simulink model "dac_spi"  (R2022a)
settings: Solver=FixedStepDiscrete  StartTime=0.0  StopTime=1000/100e6  RelTol=1e-3
libraries: hdlsllib x152, simulink x1
settings Model: DataTypeOverride=Off  Creator=ts  LastModifiedBy=ts
settings SolverCC: AlgebraicLoopSolver=TrustRegion
settings DataIOCC: LimitDataPoints=on  SaveOutput=off  SaveTime=off
settings OptimizationCC: BlockReduction=off  ConditionallyExecuteInputs=off  DefaultParameterBehavior=Inlined  LifeSpan=inf
settings DebuggingCC: AlgebraicLoopMsg=error  SingleTaskRateTransMsg=error  UnconnectedInputMsg=warning  UnconnectedOutputMsg=warning  UnconnectedLineMsg=warning  AllowSymbolicDim=off  StrictBusMsg=ErrorOnBusTreatedAsVector  SFUnexpectedBacktrackingDiag=warning  SFNoUnconditionalDefaultTransitionDiag=warning  SFExecutionAtInitializationDiag=none  SFMachineParentedDataDiag=warning  ArithmeticOperatorsInVariantConditions=warning
settings HardwareCC: ProdBitPerPointer=32  ProdBitPerSizeT=32  ProdBitPerPtrDiffT=32  ProdLargestAtomicFloat=None  ProdIntDivRoundTo=Undefined  ProdEndianess=Unspecified  ProdWordSize=32  ProdHWDeviceType=ASIC/FPGA->ASIC/FPGA  ProdEqTarget=off
settings SFSimCC: SimUseLocalCustomCode=off  CustomCodeUndefinedFunction=UseInterfaceOnly
settings RTWCC: RTWUseLocalCustomCode=off
settings CodeAppCC: StateflowObjectComments=on
settings GRTTargetCC: TargetLangStandard=C89/C90 (ANSI)
settings ConfigComp: CovScope=ReferencedModels  CovMetricSettings=dw  CovSaveCumulativeToWorkspaceVar=on  CovSaveSingleToWorkspaceVar=on  CovExternalEMLEnable=off  CovSFcnEnable=off

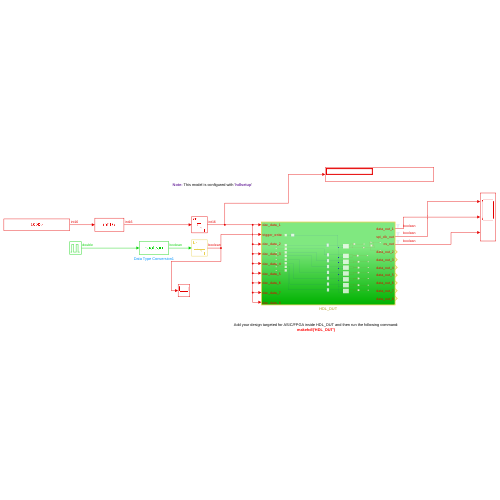
[thumbnail: Simulink's stored preview of the top-level diagram]
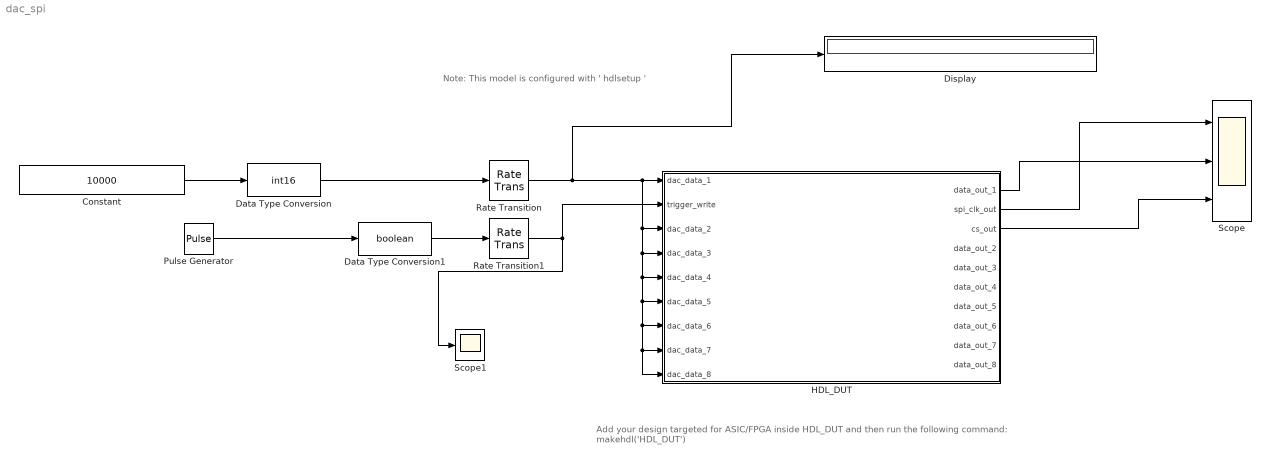
== system dac_spi ==
  note: Note: This model is configured with ' hdlsetup '
  note: Add your design targeted for ASIC/FPGA inside HDL_DUT and then run the following command:
      | makehdl('HDL_DUT')
  Constant : Constant  Value=10000  OutDataTypeStr=int16  SampleTime=1/100e6
  Data Type Conversion : DataTypeConversion  OutDataTypeStr=int16  SaturateOnIntegerOverflow=off  RndMeth=Floor
  Data Type Conversion1 : DataTypeConversion  OutDataTypeStr=boolean  SaturateOnIntegerOverflow=off  RndMeth=Floor
  Display : Display
      settings: Format=binary (Stored Integer)
  HDL_DUT : Subsystem  TreatAsAtomicUnit=on
  Pulse Generator : DiscretePulseGenerator  PulseType=Time based  Period=200/100e6  PulseWidth=10
  Rate Transition : RateTransition  OutPortSampleTime=1/100e6
  Rate Transition1 : RateTransition  OutPortSampleTime=1/100e6
  Scope : Scope  NumInputPorts=3
  Scope1 : Scope
  wires:
  Constant/1 -> Data Type Conversion/1
  HDL_DUT/1(data_out_1) -> Scope/2
  Data Type Conversion/1 -> Rate Transition/1
  Rate Transition/1 -> Display/1, HDL_DUT/9(dac_data_8), HDL_DUT/8(dac_data_7), HDL_DUT/7(dac_data_6), HDL_DUT/6(dac_data_5), HDL_DUT/5(dac_data_4), HDL_DUT/4(dac_data_3), HDL_DUT/3(dac_data_2), HDL_DUT/1(dac_data_1)
  HDL_DUT/3(cs_out) -> Scope/3
  HDL_DUT/2(spi_clk_out) -> Scope/1
  Rate Transition1/1 -> Scope1/1, HDL_DUT/2(trigger_write)
  Data Type Conversion1/1 -> Rate Transition1/1
  Pulse Generator/1 -> Data Type Conversion1/1

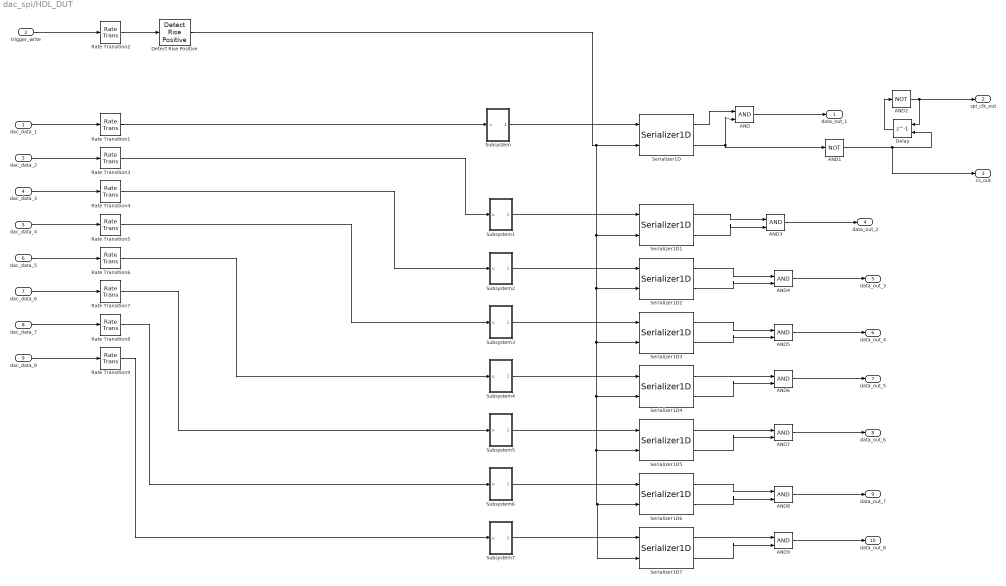
== system dac_spi/HDL_DUT ==
  dac_data_1 : Inport
  trigger_write : Inport  Port=2
  dac_data_2 : Inport  Port=3
  dac_data_3 : Inport  Port=4
  dac_data_4 : Inport  Port=5
  dac_data_5 : Inport  Port=6
  dac_data_6 : Inport  Port=7
  dac_data_7 : Inport  Port=8
  dac_data_8 : Inport  Port=9
  AND{,3..9} (8 alike) : Logic  IconShape=distinctive  AllPortsSameDT=off  OutDataTypeStr=boolean
  AND1 : Logic  Operator=NOT  IconShape=distinctive  AllPortsSameDT=off  OutDataTypeStr=boolean
  AND2 : Logic  Operator=NOT  IconShape=distinctive  AllPortsSameDT=off  OutDataTypeStr=boolean
  Delay : Delay  DelayLength=1  InitialCondition=1  ExternalReset=Level
      settings: InputPortMap=u0,r5
  Detect Rise Positive : simulink/Logic and Bit Operations/Detect Rise Positive  vinit=0  OutDataTypeStr=boolean
  Rate Transition{1..9} (9 alike) : RateTransition  OutPortSampleTime=32/100e6
  Serializer1D{,1..7} (8 alike) : hdlsllib/HDL Operations/Serializer1D  Ratio=32  IdleCycles=0  validIn=on  startOut=off  validOut=on  inputDataDimensions=-1  inputSampleTime=-1  inputSignalType=auto
      settings: SourceProductBaseCode=SL
  Subsystem : Subsystem
  Subsystem1 : Subsystem
  Subsystem2 : Subsystem
  Subsystem3 : Subsystem
  Subsystem4 : Subsystem
  Subsystem5 : Subsystem
  Subsystem6 : Subsystem
  Subsystem7 : Subsystem
  data_out_1 : Outport  VectorParamsAs1DForOutWhenUnconnected=off
  spi_clk_out : Outport  Port=2
  cs_out : Outport  Port=3
  data_out_2 : Outport  Port=4  VectorParamsAs1DForOutWhenUnconnected=off
  data_out_3 : Outport  Port=5  VectorParamsAs1DForOutWhenUnconnected=off
  data_out_4 : Outport  Port=6  VectorParamsAs1DForOutWhenUnconnected=off
  data_out_5 : Outport  Port=7  VectorParamsAs1DForOutWhenUnconnected=off
  data_out_6 : Outport  Port=8  VectorParamsAs1DForOutWhenUnconnected=off
  data_out_7 : Outport  Port=9  VectorParamsAs1DForOutWhenUnconnected=off
  data_out_8 : Outport  Port=10  VectorParamsAs1DForOutWhenUnconnected=off
  wires:
  AND/1 -> data_out_1/1
  Serializer1D/2 -> AND1/1, AND/2
  trigger_write/1 -> Rate Transition2/1
  dac_data_1/1 -> Rate Transition1/1
  Detect Rise Positive/1 -> Serializer1D7/2, Serializer1D6/2, Serializer1D5/2, Serializer1D4/2, Serializer1D3/2, Serializer1D2/2, Serializer1D1/2, Serializer1D/2
  Serializer1D/1 -> AND/1
  AND1/1 -> cs_out/1, Delay/2
  AND2/1 -> spi_clk_out/1, Delay/1
  Delay/1 -> AND2/1
  Rate Transition2/1 -> Detect Rise Positive/1
  Rate Transition1/1 -> Subsystem/1(u)
  Subsystem/1(Out1) -> Serializer1D/1
  Subsystem2/1(Out1) -> Serializer1D2/1
  Subsystem3/1(Out1) -> Serializer1D3/1
  Subsystem1/1(Out1) -> Serializer1D1/1
  dac_data_2/1 -> Rate Transition3/1
  dac_data_3/1 -> Rate Transition4/1
  dac_data_4/1 -> Rate Transition5/1
  dac_data_5/1 -> Rate Transition6/1
  dac_data_6/1 -> Rate Transition7/1
  dac_data_7/1 -> Rate Transition8/1
  dac_data_8/1 -> Rate Transition9/1
  Subsystem4/1(Out1) -> Serializer1D4/1
  Rate Transition3/1 -> Subsystem1/1(u)
  Rate Transition4/1 -> Subsystem2/1(u)
  Rate Transition5/1 -> Subsystem3/1(u)
  Rate Transition6/1 -> Subsystem4/1(u)
  Subsystem7/1(Out1) -> Serializer1D7/1
  Subsystem5/1(Out1) -> Serializer1D5/1
  Subsystem6/1(Out1) -> Serializer1D6/1
  Rate Transition7/1 -> Subsystem5/1(u)
  Rate Transition8/1 -> Subsystem6/1(u)
  Rate Transition9/1 -> Subsystem7/1(u)
  AND3/1 -> data_out_2/1
  Serializer1D1/1 -> AND3/1
  Serializer1D1/2 -> AND3/2
  AND4/1 -> data_out_3/1
  AND5/1 -> data_out_4/1
  AND6/1 -> data_out_5/1
  AND7/1 -> data_out_6/1
  AND8/1 -> data_out_7/1
  AND9/1 -> data_out_8/1
  Serializer1D2/1 -> AND4/1
  Serializer1D2/2 -> AND4/2
  Serializer1D3/1 -> AND5/1
  Serializer1D3/2 -> AND5/2
  Serializer1D4/1 -> AND6/1
  Serializer1D4/2 -> AND6/2
  Serializer1D5/1 -> AND7/1
  Serializer1D5/2 -> AND7/2
  Serializer1D6/1 -> AND8/1
  Serializer1D6/2 -> AND8/2
  Serializer1D7/1 -> AND9/1
  Serializer1D7/2 -> AND9/2

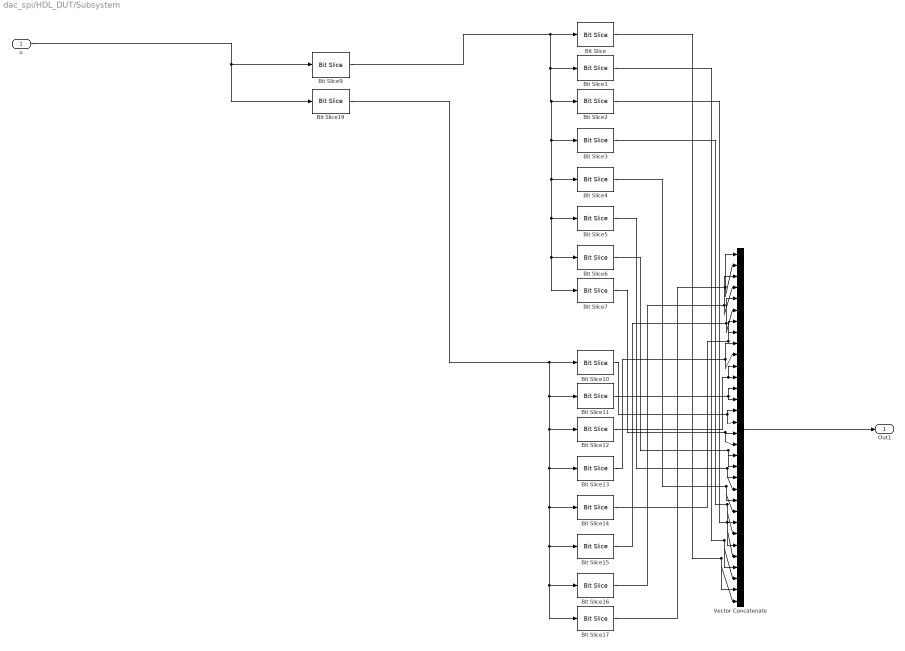
== system dac_spi/HDL_DUT/Subsystem ==
  u : Inport
  Bit Slice : hdlsllib/Logic and Bit Operations/Bit Slice  lidx=0  ridx=0
      settings: SourceProductBaseCode=SL
  Bit Slice1 : hdlsllib/Logic and Bit Operations/Bit Slice  lidx=1  ridx=1
      settings: SourceProductBaseCode=SL
  Bit Slice10 : hdlsllib/Logic and Bit Operations/Bit Slice  lidx=0  ridx=0
      settings: SourceProductBaseCode=SL
  Bit Slice11 : hdlsllib/Logic and Bit Operations/Bit Slice  lidx=1  ridx=1
      settings: SourceProductBaseCode=SL
  Bit Slice12 : hdlsllib/Logic and Bit Operations/Bit Slice  lidx=2  ridx=2
      settings: SourceProductBaseCode=SL
  Bit Slice13 : hdlsllib/Logic and Bit Operations/Bit Slice  lidx=3  ridx=3
      settings: SourceProductBaseCode=SL
  Bit Slice14 : hdlsllib/Logic and Bit Operations/Bit Slice  lidx=4  ridx=4
      settings: SourceProductBaseCode=SL
  Bit Slice15 : hdlsllib/Logic and Bit Operations/Bit Slice  lidx=5  ridx=5
      settings: SourceProductBaseCode=SL
  Bit Slice16 : hdlsllib/Logic and Bit Operations/Bit Slice  lidx=6  ridx=6
      settings: SourceProductBaseCode=SL
  Bit Slice17 : hdlsllib/Logic and Bit Operations/Bit Slice  lidx=7  ridx=7
      settings: SourceProductBaseCode=SL
  Bit Slice19 : hdlsllib/Logic and Bit Operations/Bit Slice  lidx=15  ridx=8
      settings: SourceProductBaseCode=SL
  Bit Slice2 : hdlsllib/Logic and Bit Operations/Bit Slice  lidx=2  ridx=2
      settings: SourceProductBaseCode=SL
  Bit Slice3 : hdlsllib/Logic and Bit Operations/Bit Slice  lidx=3  ridx=3
      settings: SourceProductBaseCode=SL
  Bit Slice4 : hdlsllib/Logic and Bit Operations/Bit Slice  lidx=4  ridx=4
      settings: SourceProductBaseCode=SL
  Bit Slice5 : hdlsllib/Logic and Bit Operations/Bit Slice  lidx=5  ridx=5
      settings: SourceProductBaseCode=SL
  Bit Slice6 : hdlsllib/Logic and Bit Operations/Bit Slice  lidx=6  ridx=6
      settings: SourceProductBaseCode=SL
  Bit Slice7 : hdlsllib/Logic and Bit Operations/Bit Slice  lidx=7  ridx=7
      settings: SourceProductBaseCode=SL
  Bit Slice9 : hdlsllib/Logic and Bit Operations/Bit Slice  lidx=7  ridx=0
      settings: SourceProductBaseCode=SL
  Vector Concatenate : Concatenate  NumInputs=32
  Out1 : Outport
  wires:
  Bit Slice10/1 -> Vector Concatenate/16, Vector Concatenate/15
  Bit Slice4/1 -> Vector Concatenate/24, Vector Concatenate/23
  Bit Slice6/1 -> Vector Concatenate/20, Vector Concatenate/19
  Bit Slice5/1 -> Vector Concatenate/22, Vector Concatenate/21
  u/1 -> Bit Slice19/1, Bit Slice9/1
  Bit Slice19/1 -> Bit Slice17/1, Bit Slice16/1, Bit Slice15/1, Bit Slice14/1, Bit Slice13/1, Bit Slice12/1, Bit Slice11/1, Bit Slice10/1
  Bit Slice11/1 -> Vector Concatenate/14, Vector Concatenate/13
  Bit Slice9/1 -> Bit Slice7/1, Bit Slice6/1, Bit Slice5/1, Bit Slice4/1, Bit Slice3/1, Bit Slice2/1, Bit Slice1/1, Bit Slice/1
  Bit Slice13/1 -> Vector Concatenate/10, Vector Concatenate/9
  Vector Concatenate/1 -> Out1/1
  Bit Slice7/1 -> Vector Concatenate/18, Vector Concatenate/17
  Bit Slice1/1 -> Vector Concatenate/30, Vector Concatenate/29
  Bit Slice/1 -> Vector Concatenate/32, Vector Concatenate/31
  Bit Slice17/1 -> Vector Concatenate/2, Vector Concatenate/1
  Bit Slice2/1 -> Vector Concatenate/28, Vector Concatenate/27
  Bit Slice12/1 -> Vector Concatenate/12, Vector Concatenate/11
  Bit Slice16/1 -> Vector Concatenate/4, Vector Concatenate/3
  Bit Slice14/1 -> Vector Concatenate/8, Vector Concatenate/7
  Bit Slice3/1 -> Vector Concatenate/26, Vector Concatenate/25
  Bit Slice15/1 -> Vector Concatenate/6, Vector Concatenate/5

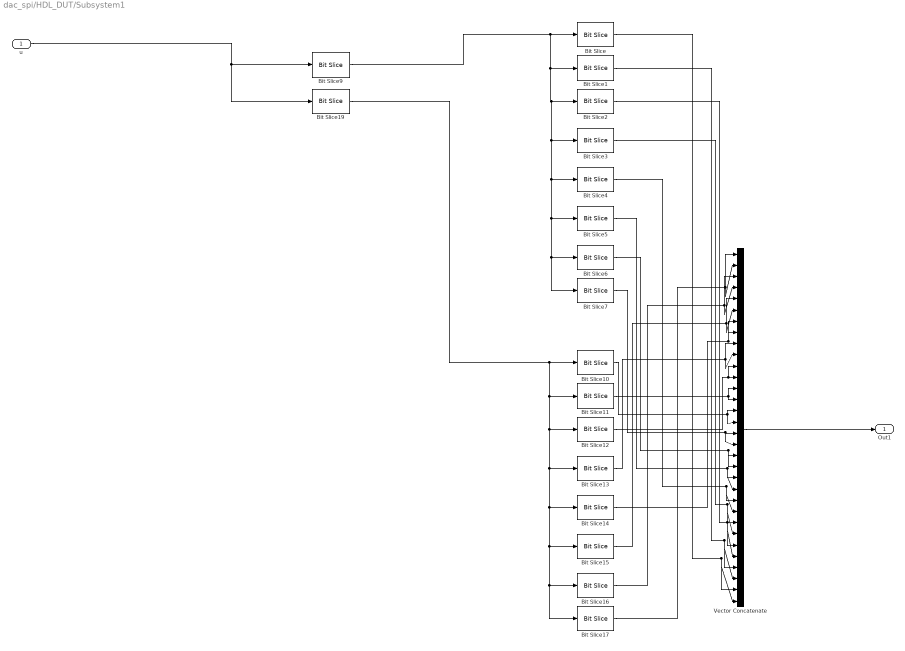
== system dac_spi/HDL_DUT/Subsystem1 ==
  u : Inport
  Bit Slice : hdlsllib/Logic and Bit Operations/Bit Slice  lidx=0  ridx=0
      settings: SourceProductBaseCode=SL
  Bit Slice1 : hdlsllib/Logic and Bit Operations/Bit Slice  lidx=1  ridx=1
      settings: SourceProductBaseCode=SL
  Bit Slice10 : hdlsllib/Logic and Bit Operations/Bit Slice  lidx=0  ridx=0
      settings: SourceProductBaseCode=SL
  Bit Slice11 : hdlsllib/Logic and Bit Operations/Bit Slice  lidx=1  ridx=1
      settings: SourceProductBaseCode=SL
  Bit Slice12 : hdlsllib/Logic and Bit Operations/Bit Slice  lidx=2  ridx=2
      settings: SourceProductBaseCode=SL
  Bit Slice13 : hdlsllib/Logic and Bit Operations/Bit Slice  lidx=3  ridx=3
      settings: SourceProductBaseCode=SL
  Bit Slice14 : hdlsllib/Logic and Bit Operations/Bit Slice  lidx=4  ridx=4
      settings: SourceProductBaseCode=SL
  Bit Slice15 : hdlsllib/Logic and Bit Operations/Bit Slice  lidx=5  ridx=5
      settings: SourceProductBaseCode=SL
  Bit Slice16 : hdlsllib/Logic and Bit Operations/Bit Slice  lidx=6  ridx=6
      settings: SourceProductBaseCode=SL
  Bit Slice17 : hdlsllib/Logic and Bit Operations/Bit Slice  lidx=7  ridx=7
      settings: SourceProductBaseCode=SL
  Bit Slice19 : hdlsllib/Logic and Bit Operations/Bit Slice  lidx=15  ridx=8
      settings: SourceProductBaseCode=SL
  Bit Slice2 : hdlsllib/Logic and Bit Operations/Bit Slice  lidx=2  ridx=2
      settings: SourceProductBaseCode=SL
  Bit Slice3 : hdlsllib/Logic and Bit Operations/Bit Slice  lidx=3  ridx=3
      settings: SourceProductBaseCode=SL
  Bit Slice4 : hdlsllib/Logic and Bit Operations/Bit Slice  lidx=4  ridx=4
      settings: SourceProductBaseCode=SL
  Bit Slice5 : hdlsllib/Logic and Bit Operations/Bit Slice  lidx=5  ridx=5
      settings: SourceProductBaseCode=SL
  Bit Slice6 : hdlsllib/Logic and Bit Operations/Bit Slice  lidx=6  ridx=6
      settings: SourceProductBaseCode=SL
  Bit Slice7 : hdlsllib/Logic and Bit Operations/Bit Slice  lidx=7  ridx=7
      settings: SourceProductBaseCode=SL
  Bit Slice9 : hdlsllib/Logic and Bit Operations/Bit Slice  lidx=7  ridx=0
      settings: SourceProductBaseCode=SL
  Vector Concatenate : Concatenate  NumInputs=32
  Out1 : Outport
  wires:
  Bit Slice15/1 -> Vector Concatenate/5, Vector Concatenate/6
  Bit Slice3/1 -> Vector Concatenate/25, Vector Concatenate/26
  Bit Slice14/1 -> Vector Concatenate/7, Vector Concatenate/8
  Bit Slice16/1 -> Vector Concatenate/3, Vector Concatenate/4
  Bit Slice12/1 -> Vector Concatenate/11, Vector Concatenate/12
  Bit Slice2/1 -> Vector Concatenate/27, Vector Concatenate/28
  Bit Slice17/1 -> Vector Concatenate/1, Vector Concatenate/2
  Bit Slice/1 -> Vector Concatenate/31, Vector Concatenate/32
  Bit Slice1/1 -> Vector Concatenate/29, Vector Concatenate/30
  Bit Slice7/1 -> Vector Concatenate/17, Vector Concatenate/18
  Vector Concatenate/1 -> Out1/1
  Bit Slice13/1 -> Vector Concatenate/9, Vector Concatenate/10
  Bit Slice9/1 -> Bit Slice/1, Bit Slice1/1, Bit Slice2/1, Bit Slice3/1, Bit Slice4/1, Bit Slice5/1, Bit Slice6/1, Bit Slice7/1
  Bit Slice11/1 -> Vector Concatenate/13, Vector Concatenate/14
  Bit Slice19/1 -> Bit Slice10/1, Bit Slice11/1, Bit Slice12/1, Bit Slice13/1, Bit Slice14/1, Bit Slice15/1, Bit Slice16/1, Bit Slice17/1
  u/1 -> Bit Slice9/1, Bit Slice19/1
  Bit Slice5/1 -> Vector Concatenate/21, Vector Concatenate/22
  Bit Slice6/1 -> Vector Concatenate/19, Vector Concatenate/20
  Bit Slice4/1 -> Vector Concatenate/23, Vector Concatenate/24
  Bit Slice10/1 -> Vector Concatenate/15, Vector Concatenate/16

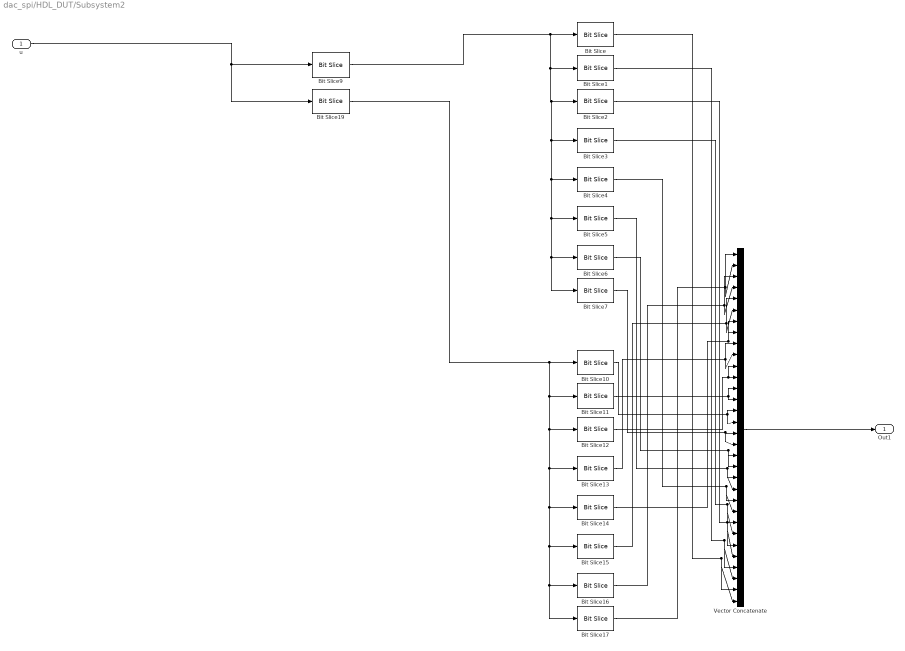
== system dac_spi/HDL_DUT/Subsystem2 ==
  u : Inport
  Bit Slice : hdlsllib/Logic and Bit Operations/Bit Slice  lidx=0  ridx=0
      settings: SourceProductBaseCode=SL
  Bit Slice1 : hdlsllib/Logic and Bit Operations/Bit Slice  lidx=1  ridx=1
      settings: SourceProductBaseCode=SL
  Bit Slice10 : hdlsllib/Logic and Bit Operations/Bit Slice  lidx=0  ridx=0
      settings: SourceProductBaseCode=SL
  Bit Slice11 : hdlsllib/Logic and Bit Operations/Bit Slice  lidx=1  ridx=1
      settings: SourceProductBaseCode=SL
  Bit Slice12 : hdlsllib/Logic and Bit Operations/Bit Slice  lidx=2  ridx=2
      settings: SourceProductBaseCode=SL
  Bit Slice13 : hdlsllib/Logic and Bit Operations/Bit Slice  lidx=3  ridx=3
      settings: SourceProductBaseCode=SL
  Bit Slice14 : hdlsllib/Logic and Bit Operations/Bit Slice  lidx=4  ridx=4
      settings: SourceProductBaseCode=SL
  Bit Slice15 : hdlsllib/Logic and Bit Operations/Bit Slice  lidx=5  ridx=5
      settings: SourceProductBaseCode=SL
  Bit Slice16 : hdlsllib/Logic and Bit Operations/Bit Slice  lidx=6  ridx=6
      settings: SourceProductBaseCode=SL
  Bit Slice17 : hdlsllib/Logic and Bit Operations/Bit Slice  lidx=7  ridx=7
      settings: SourceProductBaseCode=SL
  Bit Slice19 : hdlsllib/Logic and Bit Operations/Bit Slice  lidx=15  ridx=8
      settings: SourceProductBaseCode=SL
  Bit Slice2 : hdlsllib/Logic and Bit Operations/Bit Slice  lidx=2  ridx=2
      settings: SourceProductBaseCode=SL
  Bit Slice3 : hdlsllib/Logic and Bit Operations/Bit Slice  lidx=3  ridx=3
      settings: SourceProductBaseCode=SL
  Bit Slice4 : hdlsllib/Logic and Bit Operations/Bit Slice  lidx=4  ridx=4
      settings: SourceProductBaseCode=SL
  Bit Slice5 : hdlsllib/Logic and Bit Operations/Bit Slice  lidx=5  ridx=5
      settings: SourceProductBaseCode=SL
  Bit Slice6 : hdlsllib/Logic and Bit Operations/Bit Slice  lidx=6  ridx=6
      settings: SourceProductBaseCode=SL
  Bit Slice7 : hdlsllib/Logic and Bit Operations/Bit Slice  lidx=7  ridx=7
      settings: SourceProductBaseCode=SL
  Bit Slice9 : hdlsllib/Logic and Bit Operations/Bit Slice  lidx=7  ridx=0
      settings: SourceProductBaseCode=SL
  Vector Concatenate : Concatenate  NumInputs=32
  Out1 : Outport
  wires:
  Bit Slice10/1 -> Vector Concatenate/16, Vector Concatenate/15
  Bit Slice4/1 -> Vector Concatenate/24, Vector Concatenate/23
  Bit Slice6/1 -> Vector Concatenate/20, Vector Concatenate/19
  Bit Slice5/1 -> Vector Concatenate/22, Vector Concatenate/21
  u/1 -> Bit Slice19/1, Bit Slice9/1
  Bit Slice19/1 -> Bit Slice17/1, Bit Slice16/1, Bit Slice15/1, Bit Slice14/1, Bit Slice13/1, Bit Slice12/1, Bit Slice11/1, Bit Slice10/1
  Bit Slice11/1 -> Vector Concatenate/14, Vector Concatenate/13
  Bit Slice9/1 -> Bit Slice7/1, Bit Slice6/1, Bit Slice5/1, Bit Slice4/1, Bit Slice3/1, Bit Slice2/1, Bit Slice1/1, Bit Slice/1
  Bit Slice13/1 -> Vector Concatenate/10, Vector Concatenate/9
  Vector Concatenate/1 -> Out1/1
  Bit Slice7/1 -> Vector Concatenate/18, Vector Concatenate/17
  Bit Slice1/1 -> Vector Concatenate/30, Vector Concatenate/29
  Bit Slice/1 -> Vector Concatenate/32, Vector Concatenate/31
  Bit Slice17/1 -> Vector Concatenate/2, Vector Concatenate/1
  Bit Slice2/1 -> Vector Concatenate/28, Vector Concatenate/27
  Bit Slice12/1 -> Vector Concatenate/12, Vector Concatenate/11
  Bit Slice16/1 -> Vector Concatenate/4, Vector Concatenate/3
  Bit Slice14/1 -> Vector Concatenate/8, Vector Concatenate/7
  Bit Slice3/1 -> Vector Concatenate/26, Vector Concatenate/25
  Bit Slice15/1 -> Vector Concatenate/6, Vector Concatenate/5

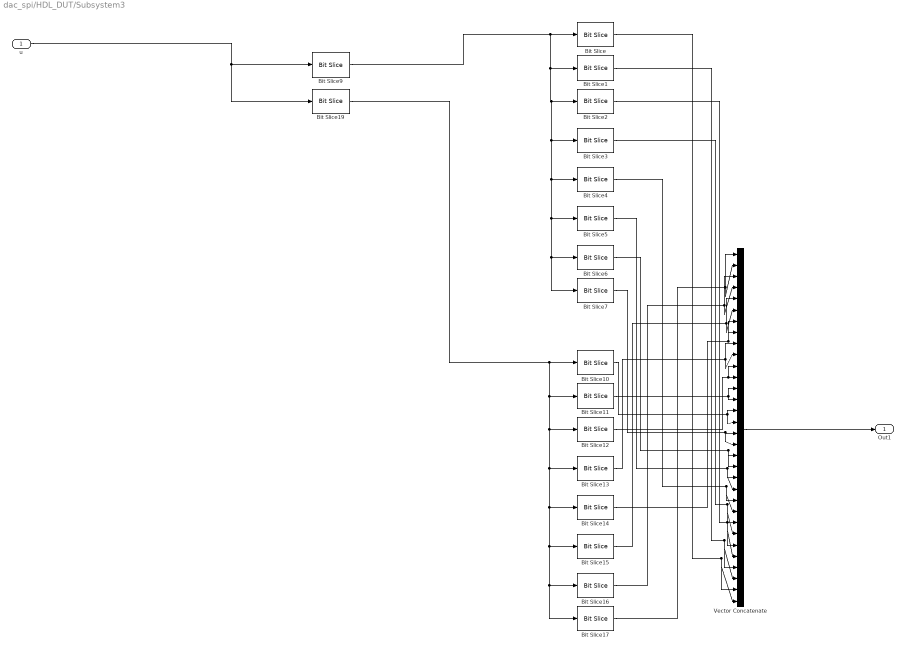
== system dac_spi/HDL_DUT/Subsystem3 ==
  u : Inport
  Bit Slice : hdlsllib/Logic and Bit Operations/Bit Slice  lidx=0  ridx=0
      settings: SourceProductBaseCode=SL
  Bit Slice1 : hdlsllib/Logic and Bit Operations/Bit Slice  lidx=1  ridx=1
      settings: SourceProductBaseCode=SL
  Bit Slice10 : hdlsllib/Logic and Bit Operations/Bit Slice  lidx=0  ridx=0
      settings: SourceProductBaseCode=SL
  Bit Slice11 : hdlsllib/Logic and Bit Operations/Bit Slice  lidx=1  ridx=1
      settings: SourceProductBaseCode=SL
  Bit Slice12 : hdlsllib/Logic and Bit Operations/Bit Slice  lidx=2  ridx=2
      settings: SourceProductBaseCode=SL
  Bit Slice13 : hdlsllib/Logic and Bit Operations/Bit Slice  lidx=3  ridx=3
      settings: SourceProductBaseCode=SL
  Bit Slice14 : hdlsllib/Logic and Bit Operations/Bit Slice  lidx=4  ridx=4
      settings: SourceProductBaseCode=SL
  Bit Slice15 : hdlsllib/Logic and Bit Operations/Bit Slice  lidx=5  ridx=5
      settings: SourceProductBaseCode=SL
  Bit Slice16 : hdlsllib/Logic and Bit Operations/Bit Slice  lidx=6  ridx=6
      settings: SourceProductBaseCode=SL
  Bit Slice17 : hdlsllib/Logic and Bit Operations/Bit Slice  lidx=7  ridx=7
      settings: SourceProductBaseCode=SL
  Bit Slice19 : hdlsllib/Logic and Bit Operations/Bit Slice  lidx=15  ridx=8
      settings: SourceProductBaseCode=SL
  Bit Slice2 : hdlsllib/Logic and Bit Operations/Bit Slice  lidx=2  ridx=2
      settings: SourceProductBaseCode=SL
  Bit Slice3 : hdlsllib/Logic and Bit Operations/Bit Slice  lidx=3  ridx=3
      settings: SourceProductBaseCode=SL
  Bit Slice4 : hdlsllib/Logic and Bit Operations/Bit Slice  lidx=4  ridx=4
      settings: SourceProductBaseCode=SL
  Bit Slice5 : hdlsllib/Logic and Bit Operations/Bit Slice  lidx=5  ridx=5
      settings: SourceProductBaseCode=SL
  Bit Slice6 : hdlsllib/Logic and Bit Operations/Bit Slice  lidx=6  ridx=6
      settings: SourceProductBaseCode=SL
  Bit Slice7 : hdlsllib/Logic and Bit Operations/Bit Slice  lidx=7  ridx=7
      settings: SourceProductBaseCode=SL
  Bit Slice9 : hdlsllib/Logic and Bit Operations/Bit Slice  lidx=7  ridx=0
      settings: SourceProductBaseCode=SL
  Vector Concatenate : Concatenate  NumInputs=32
  Out1 : Outport
  wires:
  Bit Slice15/1 -> Vector Concatenate/5, Vector Concatenate/6
  Bit Slice3/1 -> Vector Concatenate/25, Vector Concatenate/26
  Bit Slice14/1 -> Vector Concatenate/7, Vector Concatenate/8
  Bit Slice16/1 -> Vector Concatenate/3, Vector Concatenate/4
  Bit Slice12/1 -> Vector Concatenate/11, Vector Concatenate/12
  Bit Slice2/1 -> Vector Concatenate/27, Vector Concatenate/28
  Bit Slice17/1 -> Vector Concatenate/1, Vector Concatenate/2
  Bit Slice/1 -> Vector Concatenate/31, Vector Concatenate/32
  Bit Slice1/1 -> Vector Concatenate/29, Vector Concatenate/30
  Bit Slice7/1 -> Vector Concatenate/17, Vector Concatenate/18
  Vector Concatenate/1 -> Out1/1
  Bit Slice13/1 -> Vector Concatenate/9, Vector Concatenate/10
  Bit Slice9/1 -> Bit Slice/1, Bit Slice1/1, Bit Slice2/1, Bit Slice3/1, Bit Slice4/1, Bit Slice5/1, Bit Slice6/1, Bit Slice7/1
  Bit Slice11/1 -> Vector Concatenate/13, Vector Concatenate/14
  Bit Slice19/1 -> Bit Slice10/1, Bit Slice11/1, Bit Slice12/1, Bit Slice13/1, Bit Slice14/1, Bit Slice15/1, Bit Slice16/1, Bit Slice17/1
  u/1 -> Bit Slice9/1, Bit Slice19/1
  Bit Slice5/1 -> Vector Concatenate/21, Vector Concatenate/22
  Bit Slice6/1 -> Vector Concatenate/19, Vector Concatenate/20
  Bit Slice4/1 -> Vector Concatenate/23, Vector Concatenate/24
  Bit Slice10/1 -> Vector Concatenate/15, Vector Concatenate/16

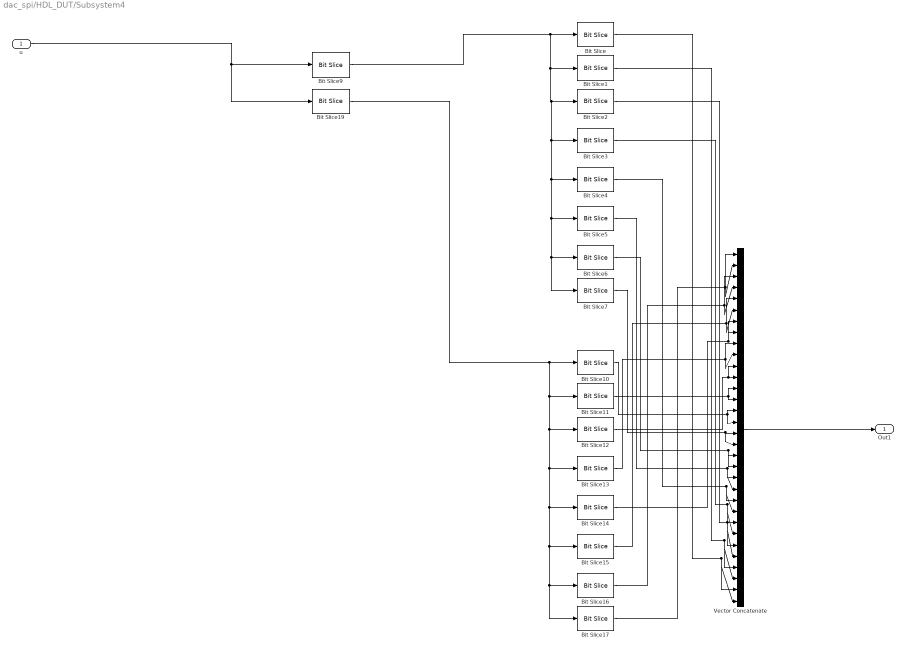
== system dac_spi/HDL_DUT/Subsystem4 ==
  u : Inport
  Bit Slice : hdlsllib/Logic and Bit Operations/Bit Slice  lidx=0  ridx=0
      settings: SourceProductBaseCode=SL
  Bit Slice1 : hdlsllib/Logic and Bit Operations/Bit Slice  lidx=1  ridx=1
      settings: SourceProductBaseCode=SL
  Bit Slice10 : hdlsllib/Logic and Bit Operations/Bit Slice  lidx=0  ridx=0
      settings: SourceProductBaseCode=SL
  Bit Slice11 : hdlsllib/Logic and Bit Operations/Bit Slice  lidx=1  ridx=1
      settings: SourceProductBaseCode=SL
  Bit Slice12 : hdlsllib/Logic and Bit Operations/Bit Slice  lidx=2  ridx=2
      settings: SourceProductBaseCode=SL
  Bit Slice13 : hdlsllib/Logic and Bit Operations/Bit Slice  lidx=3  ridx=3
      settings: SourceProductBaseCode=SL
  Bit Slice14 : hdlsllib/Logic and Bit Operations/Bit Slice  lidx=4  ridx=4
      settings: SourceProductBaseCode=SL
  Bit Slice15 : hdlsllib/Logic and Bit Operations/Bit Slice  lidx=5  ridx=5
      settings: SourceProductBaseCode=SL
  Bit Slice16 : hdlsllib/Logic and Bit Operations/Bit Slice  lidx=6  ridx=6
      settings: SourceProductBaseCode=SL
  Bit Slice17 : hdlsllib/Logic and Bit Operations/Bit Slice  lidx=7  ridx=7
      settings: SourceProductBaseCode=SL
  Bit Slice19 : hdlsllib/Logic and Bit Operations/Bit Slice  lidx=15  ridx=8
      settings: SourceProductBaseCode=SL
  Bit Slice2 : hdlsllib/Logic and Bit Operations/Bit Slice  lidx=2  ridx=2
      settings: SourceProductBaseCode=SL
  Bit Slice3 : hdlsllib/Logic and Bit Operations/Bit Slice  lidx=3  ridx=3
      settings: SourceProductBaseCode=SL
  Bit Slice4 : hdlsllib/Logic and Bit Operations/Bit Slice  lidx=4  ridx=4
      settings: SourceProductBaseCode=SL
  Bit Slice5 : hdlsllib/Logic and Bit Operations/Bit Slice  lidx=5  ridx=5
      settings: SourceProductBaseCode=SL
  Bit Slice6 : hdlsllib/Logic and Bit Operations/Bit Slice  lidx=6  ridx=6
      settings: SourceProductBaseCode=SL
  Bit Slice7 : hdlsllib/Logic and Bit Operations/Bit Slice  lidx=7  ridx=7
      settings: SourceProductBaseCode=SL
  Bit Slice9 : hdlsllib/Logic and Bit Operations/Bit Slice  lidx=7  ridx=0
      settings: SourceProductBaseCode=SL
  Vector Concatenate : Concatenate  NumInputs=32
  Out1 : Outport
  wires:
  Bit Slice15/1 -> Vector Concatenate/5, Vector Concatenate/6
  Bit Slice3/1 -> Vector Concatenate/25, Vector Concatenate/26
  Bit Slice14/1 -> Vector Concatenate/7, Vector Concatenate/8
  Bit Slice16/1 -> Vector Concatenate/3, Vector Concatenate/4
  Bit Slice12/1 -> Vector Concatenate/11, Vector Concatenate/12
  Bit Slice2/1 -> Vector Concatenate/27, Vector Concatenate/28
  Bit Slice17/1 -> Vector Concatenate/1, Vector Concatenate/2
  Bit Slice/1 -> Vector Concatenate/31, Vector Concatenate/32
  Bit Slice1/1 -> Vector Concatenate/29, Vector Concatenate/30
  Bit Slice7/1 -> Vector Concatenate/17, Vector Concatenate/18
  Vector Concatenate/1 -> Out1/1
  Bit Slice13/1 -> Vector Concatenate/9, Vector Concatenate/10
  Bit Slice9/1 -> Bit Slice/1, Bit Slice1/1, Bit Slice2/1, Bit Slice3/1, Bit Slice4/1, Bit Slice5/1, Bit Slice6/1, Bit Slice7/1
  Bit Slice11/1 -> Vector Concatenate/13, Vector Concatenate/14
  Bit Slice19/1 -> Bit Slice10/1, Bit Slice11/1, Bit Slice12/1, Bit Slice13/1, Bit Slice14/1, Bit Slice15/1, Bit Slice16/1, Bit Slice17/1
  u/1 -> Bit Slice9/1, Bit Slice19/1
  Bit Slice5/1 -> Vector Concatenate/21, Vector Concatenate/22
  Bit Slice6/1 -> Vector Concatenate/19, Vector Concatenate/20
  Bit Slice4/1 -> Vector Concatenate/23, Vector Concatenate/24
  Bit Slice10/1 -> Vector Concatenate/15, Vector Concatenate/16

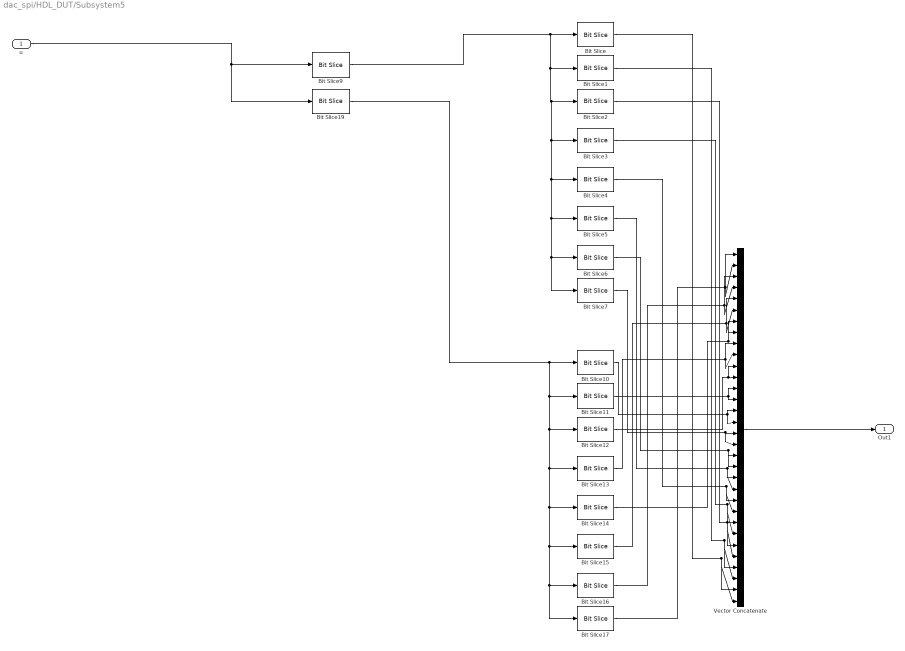
== system dac_spi/HDL_DUT/Subsystem5 ==
  u : Inport
  Bit Slice : hdlsllib/Logic and Bit Operations/Bit Slice  lidx=0  ridx=0
      settings: SourceProductBaseCode=SL
  Bit Slice1 : hdlsllib/Logic and Bit Operations/Bit Slice  lidx=1  ridx=1
      settings: SourceProductBaseCode=SL
  Bit Slice10 : hdlsllib/Logic and Bit Operations/Bit Slice  lidx=0  ridx=0
      settings: SourceProductBaseCode=SL
  Bit Slice11 : hdlsllib/Logic and Bit Operations/Bit Slice  lidx=1  ridx=1
      settings: SourceProductBaseCode=SL
  Bit Slice12 : hdlsllib/Logic and Bit Operations/Bit Slice  lidx=2  ridx=2
      settings: SourceProductBaseCode=SL
  Bit Slice13 : hdlsllib/Logic and Bit Operations/Bit Slice  lidx=3  ridx=3
      settings: SourceProductBaseCode=SL
  Bit Slice14 : hdlsllib/Logic and Bit Operations/Bit Slice  lidx=4  ridx=4
      settings: SourceProductBaseCode=SL
  Bit Slice15 : hdlsllib/Logic and Bit Operations/Bit Slice  lidx=5  ridx=5
      settings: SourceProductBaseCode=SL
  Bit Slice16 : hdlsllib/Logic and Bit Operations/Bit Slice  lidx=6  ridx=6
      settings: SourceProductBaseCode=SL
  Bit Slice17 : hdlsllib/Logic and Bit Operations/Bit Slice  lidx=7  ridx=7
      settings: SourceProductBaseCode=SL
  Bit Slice19 : hdlsllib/Logic and Bit Operations/Bit Slice  lidx=15  ridx=8
      settings: SourceProductBaseCode=SL
  Bit Slice2 : hdlsllib/Logic and Bit Operations/Bit Slice  lidx=2  ridx=2
      settings: SourceProductBaseCode=SL
  Bit Slice3 : hdlsllib/Logic and Bit Operations/Bit Slice  lidx=3  ridx=3
      settings: SourceProductBaseCode=SL
  Bit Slice4 : hdlsllib/Logic and Bit Operations/Bit Slice  lidx=4  ridx=4
      settings: SourceProductBaseCode=SL
  Bit Slice5 : hdlsllib/Logic and Bit Operations/Bit Slice  lidx=5  ridx=5
      settings: SourceProductBaseCode=SL
  Bit Slice6 : hdlsllib/Logic and Bit Operations/Bit Slice  lidx=6  ridx=6
      settings: SourceProductBaseCode=SL
  Bit Slice7 : hdlsllib/Logic and Bit Operations/Bit Slice  lidx=7  ridx=7
      settings: SourceProductBaseCode=SL
  Bit Slice9 : hdlsllib/Logic and Bit Operations/Bit Slice  lidx=7  ridx=0
      settings: SourceProductBaseCode=SL
  Vector Concatenate : Concatenate  NumInputs=32
  Out1 : Outport
  wires:
  Bit Slice10/1 -> Vector Concatenate/16, Vector Concatenate/15
  Bit Slice4/1 -> Vector Concatenate/24, Vector Concatenate/23
  Bit Slice6/1 -> Vector Concatenate/20, Vector Concatenate/19
  Bit Slice5/1 -> Vector Concatenate/22, Vector Concatenate/21
  u/1 -> Bit Slice19/1, Bit Slice9/1
  Bit Slice19/1 -> Bit Slice17/1, Bit Slice16/1, Bit Slice15/1, Bit Slice14/1, Bit Slice13/1, Bit Slice12/1, Bit Slice11/1, Bit Slice10/1
  Bit Slice11/1 -> Vector Concatenate/14, Vector Concatenate/13
  Bit Slice9/1 -> Bit Slice7/1, Bit Slice6/1, Bit Slice5/1, Bit Slice4/1, Bit Slice3/1, Bit Slice2/1, Bit Slice1/1, Bit Slice/1
  Bit Slice13/1 -> Vector Concatenate/10, Vector Concatenate/9
  Vector Concatenate/1 -> Out1/1
  Bit Slice7/1 -> Vector Concatenate/18, Vector Concatenate/17
  Bit Slice1/1 -> Vector Concatenate/30, Vector Concatenate/29
  Bit Slice/1 -> Vector Concatenate/32, Vector Concatenate/31
  Bit Slice17/1 -> Vector Concatenate/2, Vector Concatenate/1
  Bit Slice2/1 -> Vector Concatenate/28, Vector Concatenate/27
  Bit Slice12/1 -> Vector Concatenate/12, Vector Concatenate/11
  Bit Slice16/1 -> Vector Concatenate/4, Vector Concatenate/3
  Bit Slice14/1 -> Vector Concatenate/8, Vector Concatenate/7
  Bit Slice3/1 -> Vector Concatenate/26, Vector Concatenate/25
  Bit Slice15/1 -> Vector Concatenate/6, Vector Concatenate/5

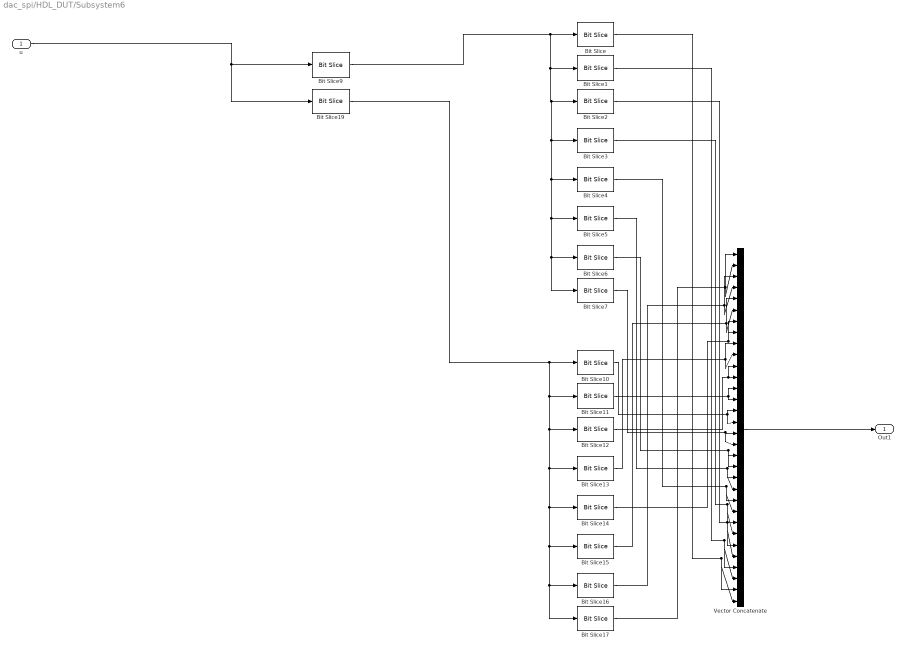
== system dac_spi/HDL_DUT/Subsystem6 ==
  u : Inport
  Bit Slice : hdlsllib/Logic and Bit Operations/Bit Slice  lidx=0  ridx=0
      settings: SourceProductBaseCode=SL
  Bit Slice1 : hdlsllib/Logic and Bit Operations/Bit Slice  lidx=1  ridx=1
      settings: SourceProductBaseCode=SL
  Bit Slice10 : hdlsllib/Logic and Bit Operations/Bit Slice  lidx=0  ridx=0
      settings: SourceProductBaseCode=SL
  Bit Slice11 : hdlsllib/Logic and Bit Operations/Bit Slice  lidx=1  ridx=1
      settings: SourceProductBaseCode=SL
  Bit Slice12 : hdlsllib/Logic and Bit Operations/Bit Slice  lidx=2  ridx=2
      settings: SourceProductBaseCode=SL
  Bit Slice13 : hdlsllib/Logic and Bit Operations/Bit Slice  lidx=3  ridx=3
      settings: SourceProductBaseCode=SL
  Bit Slice14 : hdlsllib/Logic and Bit Operations/Bit Slice  lidx=4  ridx=4
      settings: SourceProductBaseCode=SL
  Bit Slice15 : hdlsllib/Logic and Bit Operations/Bit Slice  lidx=5  ridx=5
      settings: SourceProductBaseCode=SL
  Bit Slice16 : hdlsllib/Logic and Bit Operations/Bit Slice  lidx=6  ridx=6
      settings: SourceProductBaseCode=SL
  Bit Slice17 : hdlsllib/Logic and Bit Operations/Bit Slice  lidx=7  ridx=7
      settings: SourceProductBaseCode=SL
  Bit Slice19 : hdlsllib/Logic and Bit Operations/Bit Slice  lidx=15  ridx=8
      settings: SourceProductBaseCode=SL
  Bit Slice2 : hdlsllib/Logic and Bit Operations/Bit Slice  lidx=2  ridx=2
      settings: SourceProductBaseCode=SL
  Bit Slice3 : hdlsllib/Logic and Bit Operations/Bit Slice  lidx=3  ridx=3
      settings: SourceProductBaseCode=SL
  Bit Slice4 : hdlsllib/Logic and Bit Operations/Bit Slice  lidx=4  ridx=4
      settings: SourceProductBaseCode=SL
  Bit Slice5 : hdlsllib/Logic and Bit Operations/Bit Slice  lidx=5  ridx=5
      settings: SourceProductBaseCode=SL
  Bit Slice6 : hdlsllib/Logic and Bit Operations/Bit Slice  lidx=6  ridx=6
      settings: SourceProductBaseCode=SL
  Bit Slice7 : hdlsllib/Logic and Bit Operations/Bit Slice  lidx=7  ridx=7
      settings: SourceProductBaseCode=SL
  Bit Slice9 : hdlsllib/Logic and Bit Operations/Bit Slice  lidx=7  ridx=0
      settings: SourceProductBaseCode=SL
  Vector Concatenate : Concatenate  NumInputs=32
  Out1 : Outport
  wires:
  Bit Slice15/1 -> Vector Concatenate/5, Vector Concatenate/6
  Bit Slice3/1 -> Vector Concatenate/25, Vector Concatenate/26
  Bit Slice14/1 -> Vector Concatenate/7, Vector Concatenate/8
  Bit Slice16/1 -> Vector Concatenate/3, Vector Concatenate/4
  Bit Slice12/1 -> Vector Concatenate/11, Vector Concatenate/12
  Bit Slice2/1 -> Vector Concatenate/27, Vector Concatenate/28
  Bit Slice17/1 -> Vector Concatenate/1, Vector Concatenate/2
  Bit Slice/1 -> Vector Concatenate/31, Vector Concatenate/32
  Bit Slice1/1 -> Vector Concatenate/29, Vector Concatenate/30
  Bit Slice7/1 -> Vector Concatenate/17, Vector Concatenate/18
  Vector Concatenate/1 -> Out1/1
  Bit Slice13/1 -> Vector Concatenate/9, Vector Concatenate/10
  Bit Slice9/1 -> Bit Slice/1, Bit Slice1/1, Bit Slice2/1, Bit Slice3/1, Bit Slice4/1, Bit Slice5/1, Bit Slice6/1, Bit Slice7/1
  Bit Slice11/1 -> Vector Concatenate/13, Vector Concatenate/14
  Bit Slice19/1 -> Bit Slice10/1, Bit Slice11/1, Bit Slice12/1, Bit Slice13/1, Bit Slice14/1, Bit Slice15/1, Bit Slice16/1, Bit Slice17/1
  u/1 -> Bit Slice9/1, Bit Slice19/1
  Bit Slice5/1 -> Vector Concatenate/21, Vector Concatenate/22
  Bit Slice6/1 -> Vector Concatenate/19, Vector Concatenate/20
  Bit Slice4/1 -> Vector Concatenate/23, Vector Concatenate/24
  Bit Slice10/1 -> Vector Concatenate/15, Vector Concatenate/16

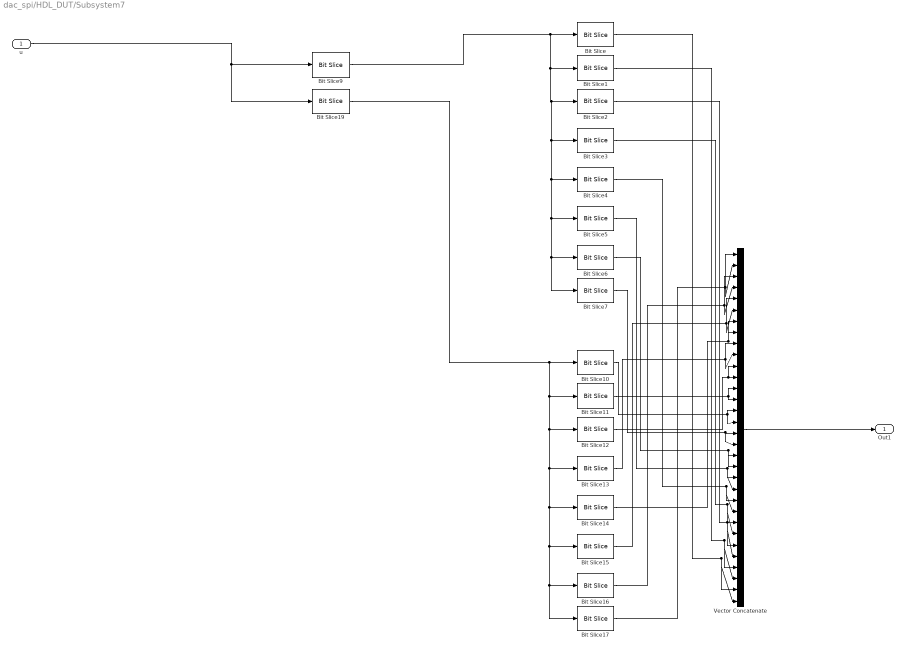
== system dac_spi/HDL_DUT/Subsystem7 ==
  u : Inport
  Bit Slice : hdlsllib/Logic and Bit Operations/Bit Slice  lidx=0  ridx=0
      settings: SourceProductBaseCode=SL
  Bit Slice1 : hdlsllib/Logic and Bit Operations/Bit Slice  lidx=1  ridx=1
      settings: SourceProductBaseCode=SL
  Bit Slice10 : hdlsllib/Logic and Bit Operations/Bit Slice  lidx=0  ridx=0
      settings: SourceProductBaseCode=SL
  Bit Slice11 : hdlsllib/Logic and Bit Operations/Bit Slice  lidx=1  ridx=1
      settings: SourceProductBaseCode=SL
  Bit Slice12 : hdlsllib/Logic and Bit Operations/Bit Slice  lidx=2  ridx=2
      settings: SourceProductBaseCode=SL
  Bit Slice13 : hdlsllib/Logic and Bit Operations/Bit Slice  lidx=3  ridx=3
      settings: SourceProductBaseCode=SL
  Bit Slice14 : hdlsllib/Logic and Bit Operations/Bit Slice  lidx=4  ridx=4
      settings: SourceProductBaseCode=SL
  Bit Slice15 : hdlsllib/Logic and Bit Operations/Bit Slice  lidx=5  ridx=5
      settings: SourceProductBaseCode=SL
  Bit Slice16 : hdlsllib/Logic and Bit Operations/Bit Slice  lidx=6  ridx=6
      settings: SourceProductBaseCode=SL
  Bit Slice17 : hdlsllib/Logic and Bit Operations/Bit Slice  lidx=7  ridx=7
      settings: SourceProductBaseCode=SL
  Bit Slice19 : hdlsllib/Logic and Bit Operations/Bit Slice  lidx=15  ridx=8
      settings: SourceProductBaseCode=SL
  Bit Slice2 : hdlsllib/Logic and Bit Operations/Bit Slice  lidx=2  ridx=2
      settings: SourceProductBaseCode=SL
  Bit Slice3 : hdlsllib/Logic and Bit Operations/Bit Slice  lidx=3  ridx=3
      settings: SourceProductBaseCode=SL
  Bit Slice4 : hdlsllib/Logic and Bit Operations/Bit Slice  lidx=4  ridx=4
      settings: SourceProductBaseCode=SL
  Bit Slice5 : hdlsllib/Logic and Bit Operations/Bit Slice  lidx=5  ridx=5
      settings: SourceProductBaseCode=SL
  Bit Slice6 : hdlsllib/Logic and Bit Operations/Bit Slice  lidx=6  ridx=6
      settings: SourceProductBaseCode=SL
  Bit Slice7 : hdlsllib/Logic and Bit Operations/Bit Slice  lidx=7  ridx=7
      settings: SourceProductBaseCode=SL
  Bit Slice9 : hdlsllib/Logic and Bit Operations/Bit Slice  lidx=7  ridx=0
      settings: SourceProductBaseCode=SL
  Vector Concatenate : Concatenate  NumInputs=32
  Out1 : Outport
  wires:
  Bit Slice15/1 -> Vector Concatenate/5, Vector Concatenate/6
  Bit Slice3/1 -> Vector Concatenate/25, Vector Concatenate/26
  Bit Slice14/1 -> Vector Concatenate/7, Vector Concatenate/8
  Bit Slice16/1 -> Vector Concatenate/3, Vector Concatenate/4
  Bit Slice12/1 -> Vector Concatenate/11, Vector Concatenate/12
  Bit Slice2/1 -> Vector Concatenate/27, Vector Concatenate/28
  Bit Slice17/1 -> Vector Concatenate/1, Vector Concatenate/2
  Bit Slice/1 -> Vector Concatenate/31, Vector Concatenate/32
  Bit Slice1/1 -> Vector Concatenate/29, Vector Concatenate/30
  Bit Slice7/1 -> Vector Concatenate/17, Vector Concatenate/18
  Vector Concatenate/1 -> Out1/1
  Bit Slice13/1 -> Vector Concatenate/9, Vector Concatenate/10
  Bit Slice9/1 -> Bit Slice/1, Bit Slice1/1, Bit Slice2/1, Bit Slice3/1, Bit Slice4/1, Bit Slice5/1, Bit Slice6/1, Bit Slice7/1
  Bit Slice11/1 -> Vector Concatenate/13, Vector Concatenate/14
  Bit Slice19/1 -> Bit Slice10/1, Bit Slice11/1, Bit Slice12/1, Bit Slice13/1, Bit Slice14/1, Bit Slice15/1, Bit Slice16/1, Bit Slice17/1
  u/1 -> Bit Slice9/1, Bit Slice19/1
  Bit Slice5/1 -> Vector Concatenate/21, Vector Concatenate/22
  Bit Slice6/1 -> Vector Concatenate/19, Vector Concatenate/20
  Bit Slice4/1 -> Vector Concatenate/23, Vector Concatenate/24
  Bit Slice10/1 -> Vector Concatenate/15, Vector Concatenate/16
